simulink model "System_composer__model_pre_alpha_V2"  (R2022b)
settings: Solver=VariableStepAuto  StartTime=0.0  StopTime=10.0  RelTol=1e-3
(part 2 of 3)

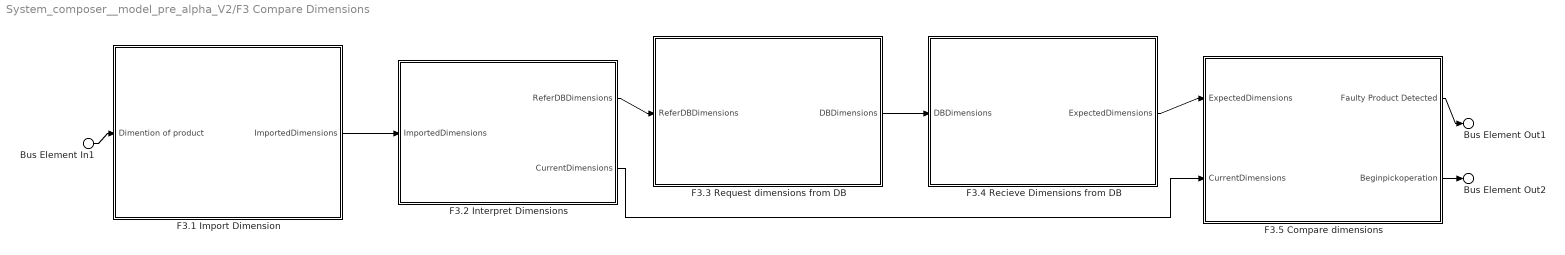
== system System_composer__model_pre_alpha_V2/F3 Compare Dimensions ==
  Bus Element In1 : Inport  PortName=Dimention of product
  F3.1 Import Dimension : Subsystem
      settings: PortSchema="{\"entries\":[{\"content\":{\"headerSize\":26,\"margin\":15,\"minimumSpacing\":25,\"sides\":[{\"content\":{\"connectorIds\":[\"In1\"]},\"type\":\"ConnectorPlacement.EquallySpacedRectSide\",\"uuid\":\"7013333b-bcb0-472a-8b4b-201a684e0f69\"},{\"content\":{\"connectorIds\":[\"Out1\"],\"side\":\"RIGHT\"},\"type\":\"ConnectorPlacement.EquallySpacedRectSide\",\"uuid\":\"4b4cc890-b976-4837-92a8-5b6c4ad3f659\"},{\"content\":{\"connectorIds\":[],\"side\":\"TOP\"},\"type\":\"ConnectorPlacement.EquallySpacedRectSide\",\"uuid\":\"d943cfaa-ae22-4a3b-a19a-c6fb5e90d8f6\"}]},\"type\":\"ConnectorPlacement.EquallySpacedConnector\",\"uuid\":\"02e5c76f-f132-4257-84b4-ea3020272a7a\"}],\"packageUris\":[\"http://schema.mathworks.com/mf0/Connector/R2020b\"],\"version\":\"1.0\"}"
  F3.2 Interpret Dimensions : Subsystem
      settings: PortSchema="{\"entries\":[{\"content\":{\"headerSize\":26,\"margin\":15,\"minimumSpacing\":25,\"sides\":[{\"content\":{\"connectorIds\":[\"In1\"]},\"type\":\"ConnectorPlacement.EquallySpacedRectSide\",\"uuid\":\"7013333b-bcb0-472a-8b4b-201a684e0f69\"},{\"content\":{\"connectorIds\":[\"Out1\",\"Out2\"],\"side\":\"RIGHT\"},\"type\":\"ConnectorPlacement.EquallySpacedRectSide\",\"uuid\":\"4b4cc890-b976-4837-92a8-5b6c4ad3f659\"},{\"content\":{\"connectorIds\":[],\"side\":\"TOP\"},\"type\":\"ConnectorPlacement.EquallySpacedRectSide\",\"uuid\":\"d943cfaa-ae22-4a3b-a19a-c6fb5e90d8f6\"}]},\"type\":\"ConnectorPlacement.EquallySpacedConnector\",\"uuid\":\"02e5c76f-f132-4257-84b4-ea3020272a7a\"}],\"packageUris\":[\"http://schema.mathworks.com/mf0/Connector/R2020b\"],\"version\":\"1.0\"}"
  F3.3 Request dimensions from DB : Subsystem
      settings: PortSchema="{\"entries\":[{\"content\":{\"headerSize\":26,\"margin\":15,\"minimumSpacing\":25,\"sides\":[{\"content\":{\"connectorIds\":[\"In1\"]},\"type\":\"ConnectorPlacement.EquallySpacedRectSide\",\"uuid\":\"7013333b-bcb0-472a-8b4b-201a684e0f69\"},{\"content\":{\"connectorIds\":[\"Out1\"],\"side\":\"RIGHT\"},\"type\":\"ConnectorPlacement.EquallySpacedRectSide\",\"uuid\":\"4b4cc890-b976-4837-92a8-5b6c4ad3f659\"},{\"content\":{\"connectorIds\":[],\"side\":\"TOP\"},\"type\":\"ConnectorPlacement.EquallySpacedRectSide\",\"uuid\":\"d943cfaa-ae22-4a3b-a19a-c6fb5e90d8f6\"}]},\"type\":\"ConnectorPlacement.EquallySpacedConnector\",\"uuid\":\"02e5c76f-f132-4257-84b4-ea3020272a7a\"}],\"packageUris\":[\"http://schema.mathworks.com/mf0/Connector/R2020b\"],\"version\":\"1.0\"}"
  F3.4 Recieve Dimensions from DB : Subsystem
      settings: PortSchema="{\"entries\":[{\"content\":{\"headerSize\":26,\"margin\":15,\"minimumSpacing\":25,\"sides\":[{\"content\":{\"connectorIds\":[\"In1\"]},\"type\":\"ConnectorPlacement.EquallySpacedRectSide\",\"uuid\":\"7013333b-bcb0-472a-8b4b-201a684e0f69\"},{\"content\":{\"connectorIds\":[\"Out1\"],\"side\":\"RIGHT\"},\"type\":\"ConnectorPlacement.EquallySpacedRectSide\",\"uuid\":\"4b4cc890-b976-4837-92a8-5b6c4ad3f659\"},{\"content\":{\"connectorIds\":[],\"side\":\"TOP\"},\"type\":\"ConnectorPlacement.EquallySpacedRectSide\",\"uuid\":\"d943cfaa-ae22-4a3b-a19a-c6fb5e90d8f6\"}]},\"type\":\"ConnectorPlacement.EquallySpacedConnector\",\"uuid\":\"02e5c76f-f132-4257-84b4-ea3020272a7a\"}],\"packageUris\":[\"http://schema.mathworks.com/mf0/Connector/R2020b\"],\"version\":\"1.0\"}"
  F3.5 Compare dimensions : Subsystem
      settings: PortSchema="{\"entries\":[{\"content\":{\"headerSize\":26,\"margin\":15,\"minimumSpacing\":25,\"sides\":[{\"content\":{\"connectorIds\":[\"In1\",\"In2\"]},\"type\":\"ConnectorPlacement.EquallySpacedRectSide\",\"uuid\":\"7013333b-bcb0-472a-8b4b-201a684e0f69\"},{\"content\":{\"connectorIds\":[\"Out1\",\"Out2\"],\"side\":\"RIGHT\"},\"type\":\"ConnectorPlacement.EquallySpacedRectSide\",\"uuid\":\"4b4cc890-b976-4837-92a8-5b6c4ad3f659\"},{\"content\":{\"connectorIds\":[],\"side\":\"TOP\"},\"type\":\"ConnectorPlacement.EquallySpacedRectSide\",\"uuid\":\"d943cfaa-ae22-4a3b-a19a-c6fb5e90d8f6\"}]},\"type\":\"ConnectorPlacement.EquallySpacedConnector\",\"uuid\":\"02e5c76f-f132-4257-84b4-ea3020272a7a\"}],\"packageUris\":[\"http://schema.mathworks.com/mf0/Connector/R2020b\"],\"version\":\"1.0\"}"
  Bus Element Out1 : Outport  PortName=Faulty Product Detected
  Bus Element Out2 : Outport  Port=2  PortName=Beiginpickoperation
  wires:
  F3.5 Compare dimensions/1(Faulty Product Detected) -> Bus Element Out1/1
  F3.3 Request dimensions from DB/1(DBDimensions) -> F3.4 Recieve Dimensions from DB/1(DBDimensions)
  F3.2 Interpret Dimensions/2(CurrentDimensions) -> F3.5 Compare dimensions/2(CurrentDimensions)
  F3.1 Import Dimension/1(ImportedDimensions) -> F3.2 Interpret Dimensions/1(ImportedDimensions)
  Bus Element In1/1 -> F3.1 Import Dimension/1(Dimention of product)
  F3.5 Compare dimensions/2(Beginpickoperation) -> Bus Element Out2/1
  F3.2 Interpret Dimensions/1(ReferDBDimensions) -> F3.3 Request dimensions from DB/1(ReferDBDimensions)
  F3.4 Recieve Dimensions from DB/1(ExpectedDimensions) -> F3.5 Compare dimensions/1(ExpectedDimensions)

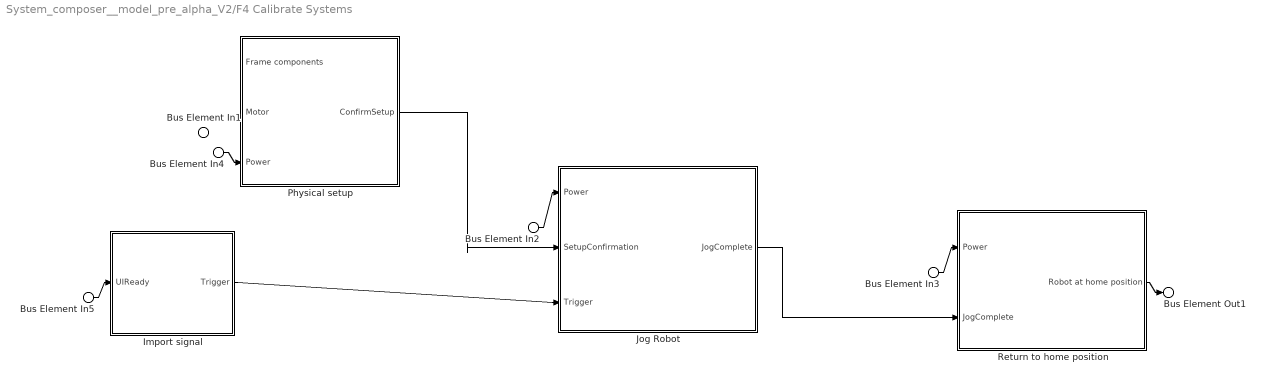
== system System_composer__model_pre_alpha_V2/F4 Calibrate Systems  ==
  Bus Element In1 : Inport  PortName=UIReady
  Bus Element In5 : Inport  PortName=UIReady
  Bus Element In2 : Inport  Port=2  PortName=Power
  Bus Element In3 : Inport  Port=2  PortName=Power
  Bus Element In4 : Inport  Port=2  PortName=Power
  Import signal : Subsystem
      settings: PortSchema="{\"entries\":[{\"content\":{\"headerSize\":26,\"margin\":15,\"minimumSpacing\":25,\"sides\":[{\"content\":{\"connectorIds\":[\"In1\"]},\"type\":\"ConnectorPlacement.EquallySpacedRectSide\",\"uuid\":\"49603a02-1e4e-4380-a56a-8f37f29afafa\"},{\"content\":{\"connectorIds\":[\"Out1\"],\"side\":\"RIGHT\"},\"type\":\"ConnectorPlacement.EquallySpacedRectSide\",\"uuid\":\"ee8e367c-9331-4580-a59d-43baf7bfc40b\"},{\"content\":{\"connectorIds\":[],\"side\":\"TOP\"},\"type\":\"ConnectorPlacement.EquallySpacedRectSide\",\"uuid\":\"fbbd32e3-58f0-4124-8dbd-de003422ef2a\"}]},\"type\":\"ConnectorPlacement.EquallySpacedConnector\",\"uuid\":\"6cb4000c-d9d6-42bd-b109-de2b1ec066aa\"}],\"packageUris\":[\"http://schema.mathworks.com/mf0/Connector/R2020b\"],\"version\":\"1.0\"}"
  Jog Robot : Subsystem
      settings: PortSchema="{\"entries\":[{\"content\":{\"headerSize\":26,\"margin\":15,\"minimumSpacing\":25,\"sides\":[{\"content\":{\"connectorIds\":[\"In1\",\"In2\",\"In3\"]},\"type\":\"ConnectorPlacement.EquallySpacedRectSide\",\"uuid\":\"49603a02-1e4e-4380-a56a-8f37f29afafa\"},{\"content\":{\"connectorIds\":[\"Out1\"],\"side\":\"RIGHT\"},\"type\":\"ConnectorPlacement.EquallySpacedRectSide\",\"uuid\":\"ee8e367c-9331-4580-a59d-43baf7bfc40b\"},{\"content\":{\"connectorIds\":[],\"side\":\"TOP\"},\"type\":\"ConnectorPlacement.EquallySpacedRectSide\",\"uuid\":\"fbbd32e3-58f0-4124-8dbd-de003422ef2a\"}]},\"type\":\"ConnectorPlacement.EquallySpacedConnector\",\"uuid\":\"6cb4000c-d9d6-42bd-b109-de2b1ec066aa\"}],\"packageUris\":[\"http://schema.mathworks.com/mf0/Connector/R2020b\"],\"version\":\"1.0\"}"
  Physical setup : Subsystem
      settings: PortSchema="{\"entries\":[{\"content\":{\"headerSize\":26,\"margin\":15,\"minimumSpacing\":25,\"sides\":[{\"content\":{\"connectorIds\":[\"In1\",\"In2\",\"In3\"]},\"type\":\"ConnectorPlacement.EquallySpacedRectSide\",\"uuid\":\"49603a02-1e4e-4380-a56a-8f37f29afafa\"},{\"content\":{\"connectorIds\":[\"Out1\"],\"side\":\"RIGHT\"},\"type\":\"ConnectorPlacement.EquallySpacedRectSide\",\"uuid\":\"ee8e367c-9331-4580-a59d-43baf7bfc40b\"},{\"content\":{\"connectorIds\":[],\"side\":\"TOP\"},\"type\":\"ConnectorPlacement.EquallySpacedRectSide\",\"uuid\":\"fbbd32e3-58f0-4124-8dbd-de003422ef2a\"}]},\"type\":\"ConnectorPlacement.EquallySpacedConnector\",\"uuid\":\"6cb4000c-d9d6-42bd-b109-de2b1ec066aa\"}],\"packageUris\":[\"http://schema.mathworks.com/mf0/Connector/R2020b\"],\"version\":\"1.0\"}"
  Return to home position : Subsystem
      settings: PortSchema="{\"entries\":[{\"content\":{\"headerSize\":26,\"margin\":15,\"minimumSpacing\":25,\"sides\":[{\"content\":{\"connectorIds\":[\"In1\",\"In2\"]},\"type\":\"ConnectorPlacement.EquallySpacedRectSide\",\"uuid\":\"49603a02-1e4e-4380-a56a-8f37f29afafa\"},{\"content\":{\"connectorIds\":[\"Out1\"],\"side\":\"RIGHT\"},\"type\":\"ConnectorPlacement.EquallySpacedRectSide\",\"uuid\":\"ee8e367c-9331-4580-a59d-43baf7bfc40b\"},{\"content\":{\"connectorIds\":[],\"side\":\"TOP\"},\"type\":\"ConnectorPlacement.EquallySpacedRectSide\",\"uuid\":\"fbbd32e3-58f0-4124-8dbd-de003422ef2a\"}]},\"type\":\"ConnectorPlacement.EquallySpacedConnector\",\"uuid\":\"6cb4000c-d9d6-42bd-b109-de2b1ec066aa\"}],\"packageUris\":[\"http://schema.mathworks.com/mf0/Connector/R2020b\"],\"version\":\"1.0\"}"
  Bus Element Out1 : Outport  PortName=ConfirmCalibration
  wires:
  Bus Element In3/1 -> Return to home position/1(Power)
  Bus Element In4/1 -> Physical setup/3(Power)
  Jog Robot/1(JogComplete) -> Return to home position/2(JogComplete)
  Physical setup/1(ConfirmSetup) -> Jog Robot/2(SetupConfirmation)
  Import signal/1(Trigger) -> Jog Robot/3(Trigger)
  Bus Element In2/1 -> Jog Robot/1(Power)
  Bus Element In5/1 -> Import signal/1(UIReady)
  Return to home position/1(Robot at home position) -> Bus Element Out1/1

== system System_composer__model_pre_alpha_V2/F9 Hold Operations ==
  Bus Element In1 : Inport  PortName=Product Not Detected
  F9.1 Pause Operation : Subsystem
      settings: PortSchema="{\"entries\":[{\"content\":{\"headerSize\":26,\"margin\":15,\"minimumSpacing\":25,\"sides\":[{\"content\":{\"connectorIds\":[\"In1\"]},\"type\":\"ConnectorPlacement.EquallySpacedRectSide\",\"uuid\":\"ee97644e-c9ff-4946-8a58-fee1d557a4ad\"},{\"content\":{\"connectorIds\":[\"Out1\"],\"side\":\"RIGHT\"},\"type\":\"ConnectorPlacement.EquallySpacedRectSide\",\"uuid\":\"e20fd496-d0ba-45f7-949d-94f28912a261\"},{\"content\":{\"connectorIds\":[],\"side\":\"TOP\"},\"type\":\"ConnectorPlacement.EquallySpacedRectSide\",\"uuid\":\"6224eb33-55c0-4770-9979-a18202099dbf\"}]},\"type\":\"ConnectorPlacement.EquallySpacedConnector\",\"uuid\":\"f8ef62f6-ad53-4f25-bdc3-ef7ca131dedb\"}],\"packageUris\":[\"http://schema.mathworks.com/mf0/Connector/R2020b\"],\"version\":\"1.0\"}"
  Conn1 : PMIOPort  Side=Left
  Bus Element Out1 : Outport  PortName=Return To Detection
  wires:
  Bus Element In1/1 -> F9.1 Pause Operation/1(Product Not Detected)
  F9.1 Pause Operation/1(Return To Detection) -> Bus Element Out1/1

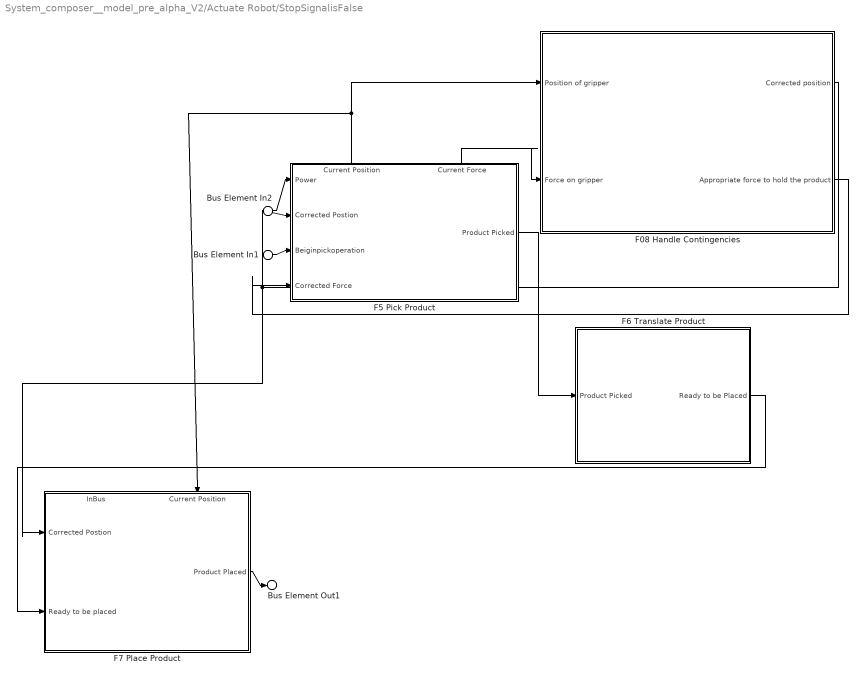
== system System_composer__model_pre_alpha_V2/Actuate Robot/StopSignalisFalse ==
  Bus Element In2 : Inport  PortName=Power
  Bus Element In1 : Inport  Port=2  PortName=Beiginpickoperation
  F08 Handle Contingencies : Subsystem
      settings: PortSchema="{\"entries\":[{\"content\":{\"headerSize\":26,\"margin\":15,\"minimumSpacing\":25,\"sides\":[{\"content\":{\"connectorIds\":[\"In1\",\"In2\"]},\"type\":\"ConnectorPlacement.EquallySpacedRectSide\",\"uuid\":\"1c117138-a6d4-4ec0-b7b8-6d1428745998\"},{\"content\":{\"connectorIds\":[\"Out1\",\"Out2\"],\"side\":\"RIGHT\"},\"type\":\"ConnectorPlacement.EquallySpacedRectSide\",\"uuid\":\"426d6ceb-18a6-42d8-9bd7-8fe69cb751f0\"},{\"content\":{\"connectorIds\":[],\"side\":\"TOP\"},\"type\":\"ConnectorPlacement.EquallySpacedRectSide\",\"uuid\":\"23012487-78cd-45b9-9306-44393710ac2e\"}]},\"type\":\"ConnectorPlacement.EquallySpacedConnector\",\"uuid\":\"f4468a7a-13e2-43af-b621-864ee5d109de\"}],\"packageUris\":[\"http://schema.mathworks.com/mf0/Connector/R2020b\"],\"version\":\"1.0\"}"
  F5 Pick Product : Subsystem
      settings: PortSchema="{\"entries\":[{\"content\":{\"headerSize\":26,\"margin\":15,\"minimumSpacing\":25,\"sides\":[{\"content\":{\"connectorIds\":[\"In1\",\"In2\",\"In3\",\"In4\"]},\"type\":\"ConnectorPlacement.EquallySpacedRectSide\",\"uuid\":\"ce520cb7-ac6b-49f5-959a-43d0066e6af8\"},{\"content\":{\"connectorIds\":[\"Out3\"],\"side\":\"RIGHT\"},\"type\":\"ConnectorPlacement.EquallySpacedRectSide\",\"uuid\":\"785c5fb5-eec3-4a9f-be3c-47cdb1865e9b\"},{\"content\":{\"connectorIds\":[\"Out1\",\"Out2\"],\"side\":\"TOP\"},\"type\":\"ConnectorPlacement.EquallySpacedRectSide\",\"uuid\":\"de1fb606-e36e-4d03-b808-745512e6c407\"}]},\"type\":\"ConnectorPlacement.EquallySpacedConnector\",\"uuid\":\"f62687dc-336d-43b3-90e2-c71aecc80de5\"}],\"packageUris\":[\"http://schema.mathworks.com/mf0/Connector/R2020b\"],\"version\":\"1.0\"}"
  F6 Translate Product : Subsystem
      settings: PortSchema="{\"entries\":[{\"content\":{\"headerSize\":26,\"margin\":15,\"minimumSpacing\":25,\"sides\":[{\"content\":{\"connectorIds\":[\"In1\"]},\"type\":\"ConnectorPlacement.EquallySpacedRectSide\",\"uuid\":\"ce520cb7-ac6b-49f5-959a-43d0066e6af8\"},{\"content\":{\"connectorIds\":[\"Out1\"],\"side\":\"RIGHT\"},\"type\":\"ConnectorPlacement.EquallySpacedRectSide\",\"uuid\":\"785c5fb5-eec3-4a9f-be3c-47cdb1865e9b\"},{\"content\":{\"connectorIds\":[],\"side\":\"TOP\"},\"type\":\"ConnectorPlacement.EquallySpacedRectSide\",\"uuid\":\"de1fb606-e36e-4d03-b808-745512e6c407\"}]},\"type\":\"ConnectorPlacement.EquallySpacedConnector\",\"uuid\":\"f62687dc-336d-43b3-90e2-c71aecc80de5\"}],\"packageUris\":[\"http://schema.mathworks.com/mf0/Connector/R2020b\"],\"version\":\"1.0\"}"
  F7 Place Product : Subsystem
      settings: PortSchema="{\"entries\":[{\"content\":{\"headerSize\":26,\"margin\":15,\"minimumSpacing\":25,\"sides\":[{\"content\":{\"connectorIds\":[\"In4\",\"In3\"]},\"type\":\"ConnectorPlacement.EquallySpacedRectSide\",\"uuid\":\"ce520cb7-ac6b-49f5-959a-43d0066e6af8\"},{\"content\":{\"connectorIds\":[\"Out1\"],\"side\":\"RIGHT\"},\"type\":\"ConnectorPlacement.EquallySpacedRectSide\",\"uuid\":\"785c5fb5-eec3-4a9f-be3c-47cdb1865e9b\"},{\"content\":{\"connectorIds\":[\"In1\",\"In2\"],\"side\":\"TOP\"},\"type\":\"ConnectorPlacement.EquallySpacedRectSide\",\"uuid\":\"de1fb606-e36e-4d03-b808-745512e6c407\"}]},\"type\":\"ConnectorPlacement.EquallySpacedConnector\",\"uuid\":\"f62687dc-336d-43b3-90e2-c71aecc80de5\"}],\"packageUris\":[\"http://schema.mathworks.com/mf0/Connector/R2020b\"],\"version\":\"1.0\"}"
  Bus Element Out1 : Outport  PortName=Product Placed
  wires:
  F6 Translate Product/1(Ready to be Placed) -> F7 Place Product/3(Ready to be placed)
  F5 Pick Product/3(Product Picked) -> F6 Translate Product/1(Product Picked)
  F5 Pick Product/1(Current Position) -> F7 Place Product/2(Current Position), F08 Handle Contingencies/1(Position of gripper)
  F08 Handle Contingencies/1(Corrected position) -> F7 Place Product/4(Corrected Postion), F5 Pick Product/2(Corrected Postion)
  F5 Pick Product/2(Current Force) -> F08 Handle Contingencies/2(Force on gripper)
  F08 Handle Contingencies/2(Appropriate force to hold the product) -> F5 Pick Product/4(Corrected Force)
  Bus Element In1/1 -> F5 Pick Product/3(Beiginpickoperation)
  Bus Element In2/1 -> F5 Pick Product/1(Power)
  F7 Place Product/1(Product Placed) -> Bus Element Out1/1

== system System_composer__model_pre_alpha_V2/Actuate Robot/StopSignalisTrue ==
  Bus Element In1 : Inport  PortName=Stop Signal
  Bus Element Out1 : Outport  PortName=NotifySTOPStatus

== system System_composer__model_pre_alpha_V2/F1 Detect Product/F1.1 Confirm System Calibration ==
  Bus Element In2 : Inport  PortName=ConfirmCalibration
  Bus Element Out1 : Outport  PortName=SystemCallibrated

== system System_composer__model_pre_alpha_V2/F1 Detect Product/F1.2 import signal ==
  Bus Element In5 : Inport  PortName=SystemCallibrated
  Bus Element In4 : Inport  Port=2  PortName=Lookforproduct
  Bus Element In3 : Inport  Port=3  PortName=Reset signal
  Bus Element Out1 : Outport  PortName=InterpretSignal

== system System_composer__model_pre_alpha_V2/F1 Detect Product/F1.3 Sense Product ==
  Bus Element In2 : Inport  PortName=Product
  Bus Element In1 : Inport  Port=2  PortName=InterpretSignal
  Bus Element Out2 : Outport  PortName=Product Detected
  Bus Element Out1 : Outport  Port=2  PortName=Count
  Bus Element Out3 : Outport  Port=3  PortName=ProductNOTdetected

== system System_composer__model_pre_alpha_V2/F10 Halt Operations/F10.1 Recieve Button Input ==
  Bus Element In1 : Inport  PortName=EmergencyStopSignal
  Bus Element Out1 : Outport  PortName=RecievedInput

== system System_composer__model_pre_alpha_V2/F10 Halt Operations/F10.2 Interpret Input ==
  Bus Element In1 : Inport  PortName=RecievedInput
  Bus Element Out1 : Outport  PortName=StopOperation

== system System_composer__model_pre_alpha_V2/F10 Halt Operations/F10.3 Stop Actuators ==
  Bus Element In1 : Inport  PortName=StopOperation
  Bus Element Out2 : Outport  PortName=NotifyOperator
  Bus Element Out1 : Outport  Port=2  PortName=Stop Signal

== system System_composer__model_pre_alpha_V2/F10 Halt Operations/F10.4 Export Signal ==
  Bus Element In1 : Inport  PortName=NotifyOperator
  Bus Element Out1 : Outport  PortName=NotifySTOP

== system System_composer__model_pre_alpha_V2/F11 Handle User Interface/F 11.1Notify user (Logout Successful) ==
  Bus Element In1 : Inport  PortName=ResetConfirm
  Bus Element Out1 : Outport  PortName=Logout Successful

== system System_composer__model_pre_alpha_V2/F11 Handle User Interface/F11.10 Monitor System Parameters ==
  Bus Element In2 : Inport  PortName=Stop Button
  Bus Element In1 : Inport  Port=2  PortName=DashboardLoaded
  Bus Element In3 : Inport  Port=3  PortName=Faulty Product Detected
  Bus Element In5 : Inport  Port=4  PortName=observeparameters
  Bus Element In4 : Inport  Port=5  PortName=Count
  Bus Element Out2 : Outport  PortName=NotifyEmergency
  Bus Element Out1 : Outport  Port=2  PortName=ShowParameters

== system System_composer__model_pre_alpha_V2/F11 Handle User Interface/F11.11 Notify User ==
  Bus Element In1 : Inport  PortName=NotifyEmergency

== system System_composer__model_pre_alpha_V2/F11 Handle User Interface/F11.12Confirm System STOP ==
  Bus Element In1 : Inport  PortName=LOGOUTConfirm
  Bus Element In2 : Inport  Port=2  PortName=STOPConfirm
  Bus Element Out1 : Outport  PortName=Resetsystem

== system System_composer__model_pre_alpha_V2/F11 Handle User Interface/F11.13 Generate STOP Signal ==
  Bus Element In1 : Inport  PortName=DBUpdated
  Bus Element Out1 : Outport  PortName=STOPoperation

== system System_composer__model_pre_alpha_V2/F11 Handle User Interface/F11.14 Update Activity Log ==
  Bus Element In1 : Inport  PortName=LogoutPrompt
  Bus Element Out1 : Outport  PortName=LOGOUTConfirm
  Bus Element Out2 : Outport  Port=2  PortName=DBUpdated

== system System_composer__model_pre_alpha_V2/F11 Handle User Interface/F11.15 Display System Parameters ==
  Bus Element In1 : Inport  PortName=ShowParameters
  Bus Element Out4 : Outport  PortName=SystemState
  Bus Element Out3 : Outport  Port=2  PortName=LogoutPrompt
  Bus Element Out2 : Outport  Port=3  PortName=observeparameters

== system System_composer__model_pre_alpha_V2/F11 Handle User Interface/F11.2 Turn ON System ==
  Bus Element In1 : Inport  PortName=Power Supply
  Bus Element Out1 : Outport  PortName=WaitforInput

== system System_composer__model_pre_alpha_V2/F11 Handle User Interface/F11.3 Recieve User Input ==
  Bus Element In1 : Inport  PortName=WaitforInput
  Bus Element In2 : Inport  Port=2  PortName=User Input
  Bus Element Out1 : Outport  PortName=ReadytoInteract

== system System_composer__model_pre_alpha_V2/F11 Handle User Interface/F11.4 Provide User Interface ==
  Bus Element In1 : Inport  PortName=ReadytoInteract
  Bus Element Out1 : Outport  PortName=VisualsReady

== system System_composer__model_pre_alpha_V2/F11 Handle User Interface/F11.5 Recieve Credentials ==
  Bus Element In1 : Inport  PortName=VisualsReady
  Bus Element In2 : Inport  Port=2  PortName=User Credentials
  Bus Element Out1 : Outport  PortName=RecievedCredentials

== system System_composer__model_pre_alpha_V2/F11 Handle User Interface/F11.6 Verify Credentials ==
  Bus Element In1 : Inport  PortName=RecievedCredentials
  Bus Element Out1 : Outport  PortName=Confirmation

== system System_composer__model_pre_alpha_V2/F11 Handle User Interface/F11.7 Confirm Login ==
  Bus Element In1 : Inport  PortName=Confirmation
  Bus Element Out2 : Outport  PortName=LOGINConfirm
  Bus Element Out1 : Outport  Port=2  PortName=OpenDashboard

== system System_composer__model_pre_alpha_V2/F11 Handle User Interface/F11.8 Provide System Dashboard ==
  Bus Element In1 : Inport  PortName=OpenDashboard
  Bus Element Out1 : Outport  PortName=DashboardLoaded

== system System_composer__model_pre_alpha_V2/F12 Reset Position/F12.1 Obtain the coordinates of home position ==
  Bus Element In1 : Inport  PortName=Product placed
  Bus Element In2 : Inport  Port=2  PortName=Log-out
  Bus Element Out1 : Outport  PortName=home position

== system System_composer__model_pre_alpha_V2/F12 Reset Position/F12.2 Go to home ==
  Bus Element In1 : Inport  PortName=home position
  Bus Element Out2 : Outport  PortName=Coordinates
  Bus Element Out1 : Outport  Port=2  PortName=power off signal

== system System_composer__model_pre_alpha_V2/F12 Reset Position/F12.3 Freeze the actuators ==
  Bus Element In1 : Inport  PortName=power off signal
  Bus Element Out1 : Outport  PortName=System ready

== system System_composer__model_pre_alpha_V2/F12 Reset Position/F12.4Hold the end effector at home position ==
  Bus Element In1 : Inport  PortName=Coordinates

== system System_composer__model_pre_alpha_V2/F2 Inspect Product/Capture image of product ==
  Bus Element In2 : Inport  PortName=Product
  Bus Element In1 : Inport  Port=2  PortName=Power
  Bus Element In3 : Inport  Port=3  PortName=Trigger
  Bus Element Out3 : Outport  PortName=ProductImage
  Bus Element Out1 : Outport  Port=2  PortName=OutBus1
  Bus Element Out2 : Outport  Port=3  PortName=OutBus

== system System_composer__model_pre_alpha_V2/F2 Inspect Product/Compute dimentions of product ==
  Bus Element In1 : Inport  PortName=Product image
  Compute dimention : Subsystem
      settings: PortSchema="{\"entries\":[{\"content\":{\"headerSize\":26,\"margin\":15,\"minimumSpacing\":25,\"sides\":[{\"content\":{\"connectorIds\":[\"In1\"]},\"type\":\"ConnectorPlacement.EquallySpacedRectSide\",\"uuid\":\"320e88d4-3d78-4d2f-ad02-b343723442c4\"},{\"content\":{\"connectorIds\":[\"Out1\"],\"side\":\"RIGHT\"},\"type\":\"ConnectorPlacement.EquallySpacedRectSide\",\"uuid\":\"09c33032-32ab-4ada-8ed8-0201f1b57dc0\"},{\"content\":{\"connectorIds\":[],\"side\":\"TOP\"},\"type\":\"ConnectorPlacement.EquallySpacedRectSide\",\"uuid\":\"2b028b26-f15f-43e2-ad75-04cde6dc5293\"}]},\"type\":\"ConnectorPlacement.EquallySpacedConnector\",\"uuid\":\"3dd2f29f-a920-492f-a094-d6d7756d0428\"}],\"packageUris\":[\"http://schema.mathworks.com/mf0/Connector/R2020b\"],\"version\":\"1.0\"}"
  get coordinates : Subsystem
      settings: PortSchema="{\"entries\":[{\"content\":{\"headerSize\":26,\"margin\":15,\"minimumSpacing\":25,\"sides\":[{\"content\":{\"connectorIds\":[\"In1\"]},\"type\":\"ConnectorPlacement.EquallySpacedRectSide\",\"uuid\":\"320e88d4-3d78-4d2f-ad02-b343723442c4\"},{\"content\":{\"connectorIds\":[\"Out1\"],\"side\":\"RIGHT\"},\"type\":\"ConnectorPlacement.EquallySpacedRectSide\",\"uuid\":\"09c33032-32ab-4ada-8ed8-0201f1b57dc0\"},{\"content\":{\"connectorIds\":[],\"side\":\"TOP\"},\"type\":\"ConnectorPlacement.EquallySpacedRectSide\",\"uuid\":\"2b028b26-f15f-43e2-ad75-04cde6dc5293\"}]},\"type\":\"ConnectorPlacement.EquallySpacedConnector\",\"uuid\":\"3dd2f29f-a920-492f-a094-d6d7756d0428\"}],\"packageUris\":[\"http://schema.mathworks.com/mf0/Connector/R2020b\"],\"version\":\"1.0\"}"
  Bus Element Out1 : Outport  PortName=Dimention of product
  wires:
  Bus Element In1/1 -> get coordinates/1(Product image)
  get coordinates/1(Coordinates) -> Compute dimention/1(Coordinates)
  Compute dimention/1(Dimention of product) -> Bus Element Out1/1

== system System_composer__model_pre_alpha_V2/F2 Inspect Product/Detect QR Code ==
  Bus Element In1 : Inport  PortName=ProductImage
  Bus Element Out1 : Outport  PortName=ExtractedQRCode

== system System_composer__model_pre_alpha_V2/F2 Inspect Product/Export Orientation ==
  Bus Element In1 : Inport  PortName=Product image
  Bus Element Out1 : Outport  PortName=ProductOrientation

== system System_composer__model_pre_alpha_V2/F2 Inspect Product/Import QR Code ==
  Bus Element In1 : Inport  PortName=ExtractedQRCOde
  Bus Element Out1 : Outport  PortName=ExportQR

== system System_composer__model_pre_alpha_V2/F2 Inspect Product/Import product ==
  Bus Element In1 : Inport  PortName=Product
  Bus Element Out1 : Outport  PortName=OutBus

== system System_composer__model_pre_alpha_V2/F2 Inspect Product/Import signal ==
  Bus Element In1 : Inport  PortName=Detection signal
  Bus Element Out1 : Outport  PortName=Trigger

== system System_composer__model_pre_alpha_V2/F2 Inspect Product/Record position of Product ==
  Bus Element In1 : Inport  PortName=Product image
  Bus Element Out1 : Outport  PortName=ProductPosition

== system System_composer__model_pre_alpha_V2/F3 Compare Dimensions/F3.1 Import Dimension ==
  Bus Element In1 : Inport  PortName=Dimention of product
  Bus Element Out1 : Outport  PortName=ImportedDimensions

== system System_composer__model_pre_alpha_V2/F3 Compare Dimensions/F3.2 Interpret Dimensions ==
  Bus Element In1 : Inport  PortName=ImportedDimensions
  Bus Element Out1 : Outport  PortName=ReferDBDimensions
  Bus Element Out2 : Outport  Port=2  PortName=CurrentDimensions

== system System_composer__model_pre_alpha_V2/F3 Compare Dimensions/F3.3 Request dimensions from DB ==
  Bus Element In1 : Inport  PortName=ReferDBDimensions
  Bus Element Out1 : Outport  PortName=DBDimensions

== system System_composer__model_pre_alpha_V2/F3 Compare Dimensions/F3.4 Recieve Dimensions from DB ==
  Bus Element In1 : Inport  PortName=DBDimensions
  Bus Element Out1 : Outport  PortName=ExpectedDimensions

== system System_composer__model_pre_alpha_V2/F3 Compare Dimensions/F3.5 Compare dimensions ==
  Bus Element In2 : Inport  PortName=ExpectedDimensions
  Bus Element In1 : Inport  Port=2  PortName=CurrentDimensions
  Bus Element Out1 : Outport  PortName=Faulty Product Detected
  Bus Element Out2 : Outport  Port=2  PortName=Beginpickoperation

== system System_composer__model_pre_alpha_V2/F4 Calibrate Systems /Import signal ==
  Bus Element In1 : Inport  PortName=UIReady
  Bus Element Out1 : Outport  PortName=Trigger

== system System_composer__model_pre_alpha_V2/F4 Calibrate Systems /Jog Robot ==
  Bus Element In1 : Inport  PortName=Power
  Bus Element In2 : Inport  Port=2  PortName=SetupConfirmation
  Bus Element In3 : Inport  Port=3  PortName=Trigger
  Bus Element Out1 : Outport  PortName=JogComplete

== system System_composer__model_pre_alpha_V2/F4 Calibrate Systems /Physical setup ==
  Bus Element In1 : Inport  PortName=Frame components
  Bus Element In2 : Inport  Port=2  PortName=Motor
  Bus Element In3 : Inport  Port=3  PortName=Power
  Frame setup : Subsystem
      settings: PortSchema="{\"entries\":[{\"content\":{\"headerSize\":26,\"margin\":15,\"minimumSpacing\":25,\"sides\":[{\"content\":{\"connectorIds\":[\"In1\"]},\"type\":\"ConnectorPlacement.EquallySpacedRectSide\",\"uuid\":\"49603a02-1e4e-4380-a56a-8f37f29afafa\"},{\"content\":{\"connectorIds\":[\"Out1\"],\"side\":\"RIGHT\"},\"type\":\"ConnectorPlacement.EquallySpacedRectSide\",\"uuid\":\"ee8e367c-9331-4580-a59d-43baf7bfc40b\"},{\"content\":{\"connectorIds\":[],\"side\":\"TOP\"},\"type\":\"ConnectorPlacement.EquallySpacedRectSide\",\"uuid\":\"fbbd32e3-58f0-4124-8dbd-de003422ef2a\"}]},\"type\":\"ConnectorPlacement.EquallySpacedConnector\",\"uuid\":\"6cb4000c-d9d6-42bd-b109-de2b1ec066aa\"}],\"packageUris\":[\"http://schema.mathworks.com/mf0/Connector/R2020b\"],\"version\":\"1.0\"}"
  Motor setup : Subsystem
      settings: PortSchema="{\"entries\":[{\"content\":{\"headerSize\":26,\"margin\":15,\"minimumSpacing\":25,\"sides\":[{\"content\":{\"connectorIds\":[\"In1\",\"In2\"]},\"type\":\"ConnectorPlacement.EquallySpacedRectSide\",\"uuid\":\"49603a02-1e4e-4380-a56a-8f37f29afafa\"},{\"content\":{\"connectorIds\":[\"Out1\"],\"side\":\"RIGHT\"},\"type\":\"ConnectorPlacement.EquallySpacedRectSide\",\"uuid\":\"ee8e367c-9331-4580-a59d-43baf7bfc40b\"},{\"content\":{\"connectorIds\":[],\"side\":\"TOP\"},\"type\":\"ConnectorPlacement.EquallySpacedRectSide\",\"uuid\":\"fbbd32e3-58f0-4124-8dbd-de003422ef2a\"}]},\"type\":\"ConnectorPlacement.EquallySpacedConnector\",\"uuid\":\"6cb4000c-d9d6-42bd-b109-de2b1ec066aa\"}],\"packageUris\":[\"http://schema.mathworks.com/mf0/Connector/R2020b\"],\"version\":\"1.0\"}"
  Power upset : Subsystem
      settings: PortSchema="{\"entries\":[{\"content\":{\"headerSize\":26,\"margin\":15,\"minimumSpacing\":25,\"sides\":[{\"content\":{\"connectorIds\":[\"In1\",\"In2\"]},\"type\":\"ConnectorPlacement.EquallySpacedRectSide\",\"uuid\":\"49603a02-1e4e-4380-a56a-8f37f29afafa\"},{\"content\":{\"connectorIds\":[\"Out1\"],\"side\":\"RIGHT\"},\"type\":\"ConnectorPlacement.EquallySpacedRectSide\",\"uuid\":\"ee8e367c-9331-4580-a59d-43baf7bfc40b\"},{\"content\":{\"connectorIds\":[],\"side\":\"TOP\"},\"type\":\"ConnectorPlacement.EquallySpacedRectSide\",\"uuid\":\"fbbd32e3-58f0-4124-8dbd-de003422ef2a\"}]},\"type\":\"ConnectorPlacement.EquallySpacedConnector\",\"uuid\":\"6cb4000c-d9d6-42bd-b109-de2b1ec066aa\"}],\"packageUris\":[\"http://schema.mathworks.com/mf0/Connector/R2020b\"],\"version\":\"1.0\"}"
  Bus Element Out1 : Outport  PortName=ConfirmSetup
  wires:
  Bus Element In1/1 -> Frame setup/1(Frame components)
  Frame setup/1(Frame) -> Motor setup/1(Frame)
  Motor setup/1(Frame and motor setup) -> Power upset/2(Frame and motor setup)
  Bus Element In2/1 -> Motor setup/2(Motor)
  Bus Element In3/1 -> Power upset/1(Power)
  Power upset/1(Physical setup) -> Bus Element Out1/1

== system System_composer__model_pre_alpha_V2/F4 Calibrate Systems /Return to home position ==
  Bus Element In2 : Inport  PortName=Power
  Bus Element In1 : Inport  Port=2  PortName=JogComplete
  Bus Element Out1 : Outport  PortName=Robot at home position

== system System_composer__model_pre_alpha_V2/F9 Hold Operations/F9.1 Pause Operation ==
  Bus Element In1 : Inport  PortName=Product Not Detected
  Bus Element Out1 : Outport  PortName=Return To Detection

== system System_composer__model_pre_alpha_V2/Actuate Robot/StopSignalisFalse/F08 Handle Contingencies ==
  In Bus Element : Inport  PortName=Position of gripper
  In Bus Element1 : Inport  Port=2  PortName=Force on gripper
  Check Pick Position : Subsystem  Variant=on  VariantControlMode=label  LabelModeActiveChoice=true
      settings: PortSchema="{\"entries\":[{\"content\":{\"headerSize\":38,\"margin\":15,\"minimumSpacing\":25,\"sides\":[{\"content\":{\"connectorIds\":[\"In1\"]},\"type\":\"ConnectorPlacement.EquallySpacedRectSide\",\"uuid\":\"82248304-a162-48ca-a47b-1ca98baf0c4b\"},{\"content\":{\"connectorIds\":[\"Out1\"],\"side\":\"RIGHT\"},\"type\":\"ConnectorPlacement.EquallySpacedRectSide\",\"uuid\":\"4a71fcf9-75ca-4fc2-a495-265b9c18be6e\"},{\"content\":{\"connectorIds\":[],\"side\":\"TOP\"},\"type\":\"ConnectorPlacement.EquallySpacedRectSide\",\"uuid\":\"a8916134-5d81-43cb-b01e-b135fd95b202\"}]},\"type\":\"ConnectorPlacement.EquallySpacedConnector\",\"uuid\":\"0453f589-d612-429d-a4fd-aaf4ba456e8c\"}],\"packageUris\":[\"http://schema.mathworks.com/mf0/Connector/R2020b\"],\"version\":\"1.0\"}"
  F8.1Weak force on the product : Subsystem
      settings: PortSchema="{\"entries\":[{\"content\":{\"headerSize\":26,\"margin\":15,\"minimumSpacing\":25,\"sides\":[{\"content\":{\"connectorIds\":[\"In1\"]},\"type\":\"ConnectorPlacement.EquallySpacedRectSide\",\"uuid\":\"cfa9a458-ccb1-4b4b-9223-cdb6aaef5fc4\"},{\"content\":{\"connectorIds\":[\"Out1\"],\"side\":\"RIGHT\"},\"type\":\"ConnectorPlacement.EquallySpacedRectSide\",\"uuid\":\"f9e6f688-270f-46a5-8c07-32c6831cf3d3\"},{\"content\":{\"connectorIds\":[],\"side\":\"TOP\"},\"type\":\"ConnectorPlacement.EquallySpacedRectSide\",\"uuid\":\"2fcd258a-a10a-44a0-bcb2-682252ae81b0\"}]},\"type\":\"ConnectorPlacement.EquallySpacedConnector\",\"uuid\":\"80e45476-3fa2-42b9-aef1-d9f502108577\"}],\"packageUris\":[\"http://schema.mathworks.com/mf0/Connector/R2020b\"],\"version\":\"1.0\"}"
  Out Bus Element1 : Outport  PortName=Corrected position
  Out Bus Element : Outport  Port=2  PortName=Appropriate force to hold the product
  wires:
  In Bus Element1/1 -> F8.1Weak force on the product/1(Force on gripper)
  In Bus Element/1 -> Check Pick Position/1(Position of gripper)
  Check Pick Position/1(Corrected position) -> Out Bus Element1/1
  F8.1Weak force on the product/1(Appropriate force) -> Out Bus Element/1

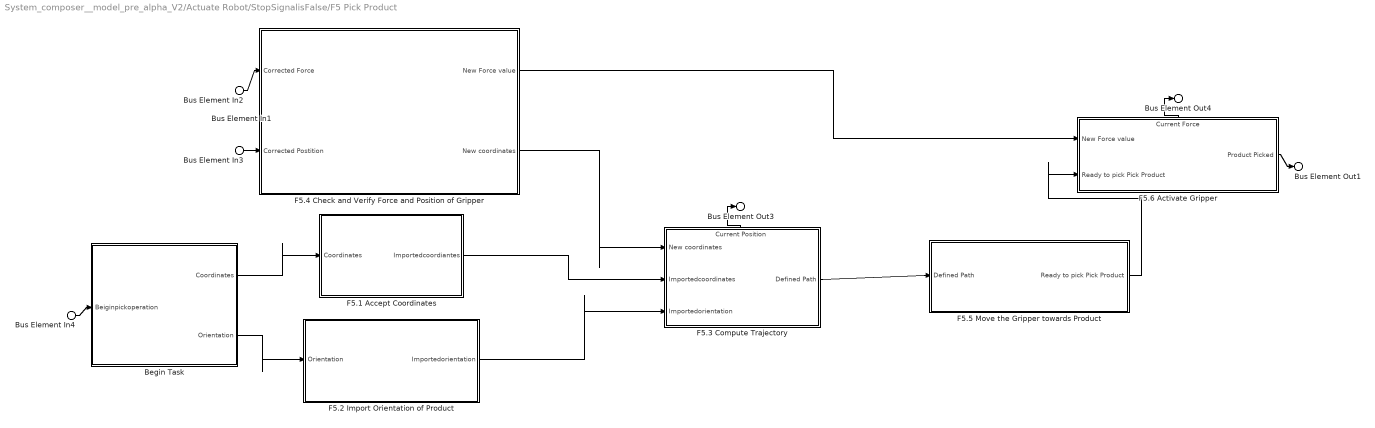
== system System_composer__model_pre_alpha_V2/Actuate Robot/StopSignalisFalse/F5 Pick Product ==
  Bus Element In1 : Inport  PortName=Power
  Bus Element In2 : Inport  Port=2  PortName=Corrected Postion
  Bus Element In4 : Inport  Port=3  PortName=Beiginpickoperation
  Bus Element In3 : Inport  Port=4  PortName=Corrected Force
  Begin Task : Subsystem
      settings: PortSchema="{\"entries\":[{\"content\":{\"headerSize\":26,\"margin\":15,\"minimumSpacing\":25,\"sides\":[{\"content\":{\"connectorIds\":[\"In1\"]},\"type\":\"ConnectorPlacement.EquallySpacedRectSide\",\"uuid\":\"ae240f5f-39ed-41a3-b9a8-bf2f33b986be\"},{\"content\":{\"connectorIds\":[\"Out1\",\"Out2\"],\"side\":\"RIGHT\"},\"type\":\"ConnectorPlacement.EquallySpacedRectSide\",\"uuid\":\"44ba199a-fd12-4621-8565-f3f1adedec4a\"},{\"content\":{\"connectorIds\":[],\"side\":\"TOP\"},\"type\":\"ConnectorPlacement.EquallySpacedRectSide\",\"uuid\":\"41d301d8-0f91-4ed1-b07b-750dd04e1ae2\"}]},\"type\":\"ConnectorPlacement.EquallySpacedConnector\",\"uuid\":\"8d081691-644b-416f-87ea-d7e0a52b2ce6\"}],\"packageUris\":[\"http://schema.mathworks.com/mf0/Connector/R2020b\"],\"version\":\"1.0\"}"
  F5.1 Accept Coordinates : Subsystem
      settings: PortSchema="{\"entries\":[{\"content\":{\"headerSize\":26,\"margin\":15,\"minimumSpacing\":25,\"sides\":[{\"content\":{\"connectorIds\":[\"In1\"]},\"type\":\"ConnectorPlacement.EquallySpacedRectSide\",\"uuid\":\"ce520cb7-ac6b-49f5-959a-43d0066e6af8\"},{\"content\":{\"connectorIds\":[\"Out1\"],\"side\":\"RIGHT\"},\"type\":\"ConnectorPlacement.EquallySpacedRectSide\",\"uuid\":\"785c5fb5-eec3-4a9f-be3c-47cdb1865e9b\"},{\"content\":{\"connectorIds\":[],\"side\":\"TOP\"},\"type\":\"ConnectorPlacement.EquallySpacedRectSide\",\"uuid\":\"de1fb606-e36e-4d03-b808-745512e6c407\"}]},\"type\":\"ConnectorPlacement.EquallySpacedConnector\",\"uuid\":\"f62687dc-336d-43b3-90e2-c71aecc80de5\"}],\"packageUris\":[\"http://schema.mathworks.com/mf0/Connector/R2020b\"],\"version\":\"1.0\"}"
  F5.2 Import Orientation of Product : Subsystem
      settings: PortSchema="{\"entries\":[{\"content\":{\"headerSize\":26,\"margin\":15,\"minimumSpacing\":25,\"sides\":[{\"content\":{\"connectorIds\":[\"In1\"]},\"type\":\"ConnectorPlacement.EquallySpacedRectSide\",\"uuid\":\"ce520cb7-ac6b-49f5-959a-43d0066e6af8\"},{\"content\":{\"connectorIds\":[\"Out1\"],\"side\":\"RIGHT\"},\"type\":\"ConnectorPlacement.EquallySpacedRectSide\",\"uuid\":\"785c5fb5-eec3-4a9f-be3c-47cdb1865e9b\"},{\"content\":{\"connectorIds\":[],\"side\":\"TOP\"},\"type\":\"ConnectorPlacement.EquallySpacedRectSide\",\"uuid\":\"de1fb606-e36e-4d03-b808-745512e6c407\"}]},\"type\":\"ConnectorPlacement.EquallySpacedConnector\",\"uuid\":\"f62687dc-336d-43b3-90e2-c71aecc80de5\"}],\"packageUris\":[\"http://schema.mathworks.com/mf0/Connector/R2020b\"],\"version\":\"1.0\"}"
  F5.3 Compute Trajectory : Subsystem
      settings: PortSchema="{\"entries\":[{\"content\":{\"headerSize\":26,\"margin\":15,\"minimumSpacing\":25,\"sides\":[{\"content\":{\"connectorIds\":[\"In1\",\"In2\",\"In3\"]},\"type\":\"ConnectorPlacement.EquallySpacedRectSide\",\"uuid\":\"ce520cb7-ac6b-49f5-959a-43d0066e6af8\"},{\"content\":{\"connectorIds\":[\"Out2\"],\"side\":\"RIGHT\"},\"type\":\"ConnectorPlacement.EquallySpacedRectSide\",\"uuid\":\"785c5fb5-eec3-4a9f-be3c-47cdb1865e9b\"},{\"content\":{\"connectorIds\":[\"Out1\"],\"side\":\"TOP\"},\"type\":\"ConnectorPlacement.EquallySpacedRectSide\",\"uuid\":\"de1fb606-e36e-4d03-b808-745512e6c407\"}]},\"type\":\"ConnectorPlacement.EquallySpacedConnector\",\"uuid\":\"f62687dc-336d-43b3-90e2-c71aecc80de5\"}],\"packageUris\":[\"http://schema.mathworks.com/mf0/Connector/R2020b\"],\"version\":\"1.0\"}"
  F5.4 Check and Verify Force and Position of Gripper : Subsystem
      settings: PortSchema="{\"entries\":[{\"content\":{\"headerSize\":26,\"margin\":15,\"minimumSpacing\":25,\"sides\":[{\"content\":{\"connectorIds\":[\"In1\",\"In2\"]},\"type\":\"ConnectorPlacement.EquallySpacedRectSide\",\"uuid\":\"ce520cb7-ac6b-49f5-959a-43d0066e6af8\"},{\"content\":{\"connectorIds\":[\"Out1\",\"Out2\"],\"side\":\"RIGHT\"},\"type\":\"ConnectorPlacement.EquallySpacedRectSide\",\"uuid\":\"785c5fb5-eec3-4a9f-be3c-47cdb1865e9b\"},{\"content\":{\"connectorIds\":[],\"side\":\"TOP\"},\"type\":\"ConnectorPlacement.EquallySpacedRectSide\",\"uuid\":\"de1fb606-e36e-4d03-b808-745512e6c407\"},{\"content\":{\"connectorIds\":[],\"side\":\"BOTTOM\"},\"type\":\"ConnectorPlacement.EquallySpacedRectSide\",\"uuid\":\"853ec498-094f-4e09-abd5-bb70086bab7d\"}]},\"type\":\"ConnectorPlacement.EquallySpacedConnector\",\"uuid\":\"f62687dc-336d-43b3-90e2-c71aecc80de5\"}],\"packageUris\":[\"http://schema.mathworks.com/mf0/Connector/R2020b\"],\"version\":\"1.0\"}"
  F5.5 Move the Gripper towards Product : Subsystem
      settings: PortSchema="{\"entries\":[{\"content\":{\"headerSize\":26,\"margin\":15,\"minimumSpacing\":25,\"sides\":[{\"content\":{\"connectorIds\":[\"In1\"]},\"type\":\"ConnectorPlacement.EquallySpacedRectSide\",\"uuid\":\"ce520cb7-ac6b-49f5-959a-43d0066e6af8\"},{\"content\":{\"connectorIds\":[\"Out1\"],\"side\":\"RIGHT\"},\"type\":\"ConnectorPlacement.EquallySpacedRectSide\",\"uuid\":\"785c5fb5-eec3-4a9f-be3c-47cdb1865e9b\"},{\"content\":{\"connectorIds\":[],\"side\":\"TOP\"},\"type\":\"ConnectorPlacement.EquallySpacedRectSide\",\"uuid\":\"de1fb606-e36e-4d03-b808-745512e6c407\"}]},\"type\":\"ConnectorPlacement.EquallySpacedConnector\",\"uuid\":\"f62687dc-336d-43b3-90e2-c71aecc80de5\"}],\"packageUris\":[\"http://schema.mathworks.com/mf0/Connector/R2020b\"],\"version\":\"1.0\"}"
  F5.6 Activate Gripper : Subsystem
      settings: PortSchema="{\"entries\":[{\"content\":{\"headerSize\":26,\"margin\":15,\"minimumSpacing\":25,\"sides\":[{\"content\":{\"connectorIds\":[\"In1\",\"In2\"]},\"type\":\"ConnectorPlacement.EquallySpacedRectSide\",\"uuid\":\"ce520cb7-ac6b-49f5-959a-43d0066e6af8\"},{\"content\":{\"connectorIds\":[\"Out2\"],\"side\":\"RIGHT\"},\"type\":\"ConnectorPlacement.EquallySpacedRectSide\",\"uuid\":\"785c5fb5-eec3-4a9f-be3c-47cdb1865e9b\"},{\"content\":{\"connectorIds\":[\"Out1\"],\"side\":\"TOP\"},\"type\":\"ConnectorPlacement.EquallySpacedRectSide\",\"uuid\":\"de1fb606-e36e-4d03-b808-745512e6c407\"}]},\"type\":\"ConnectorPlacement.EquallySpacedConnector\",\"uuid\":\"f62687dc-336d-43b3-90e2-c71aecc80de5\"}],\"packageUris\":[\"http://schema.mathworks.com/mf0/Connector/R2020b\"],\"version\":\"1.0\"}"
  Bus Element Out3 : Outport  PortName=Current Position
  Bus Element Out4 : Outport  Port=2  PortName=Current Force
  Bus Element Out1 : Outport  Port=3  PortName=Product Picked
  wires:
  F5.4 Check and Verify Force and Position of Gripper/1(New Force value) -> F5.6 Activate Gripper/1(New Force value)
  Bus Element In2/1 -> F5.4 Check and Verify Force and Position of Gripper/1(Corrected Force)
  Bus Element In3/1 -> F5.4 Check and Verify Force and Position of Gripper/2(Corrected Postition)
  F5.1 Accept Coordinates/1(Importedcoordiantes) -> F5.3 Compute Trajectory/2(Importedcoordinates)
  F5.4 Check and Verify Force and Position of Gripper/2(New coordinates) -> F5.3 Compute Trajectory/1(New coordinates)
  F5.2 Import Orientation of Product/1(Importedorientation) -> F5.3 Compute Trajectory/3(Importedorientation)
  F5.3 Compute Trajectory/2(Defined Path) -> F5.5 Move the Gripper towards Product/1(Defined Path)
  F5.5 Move the Gripper towards Product/1(Ready to pick Pick Product) -> F5.6 Activate Gripper/2(Ready to pick Pick Product)
  F5.6 Activate Gripper/2(Product Picked) -> Bus Element Out1/1
  Begin Task/1(Coordinates) -> F5.1 Accept Coordinates/1(Coordinates)
  Begin Task/2(Orientation) -> F5.2 Import Orientation of Product/1(Orientation)
  Bus Element In4/1 -> Begin Task/1(Beiginpickoperation)
  F5.3 Compute Trajectory/1(Current Position) -> Bus Element Out3/1
  F5.6 Activate Gripper/1(Current Force) -> Bus Element Out4/1

== system System_composer__model_pre_alpha_V2/Actuate Robot/StopSignalisFalse/F6 Translate Product ==
  Bus Element In1 : Inport  PortName=Product Picked
  F6.1 Move : Subsystem
      settings: PortSchema="{\"entries\":[{\"content\":{\"headerSize\":26,\"margin\":15,\"minimumSpacing\":25,\"sides\":[{\"content\":{\"connectorIds\":[\"In1\"]},\"type\":\"ConnectorPlacement.EquallySpacedRectSide\",\"uuid\":\"ce520cb7-ac6b-49f5-959a-43d0066e6af8\"},{\"content\":{\"connectorIds\":[\"Out1\"],\"side\":\"RIGHT\"},\"type\":\"ConnectorPlacement.EquallySpacedRectSide\",\"uuid\":\"785c5fb5-eec3-4a9f-be3c-47cdb1865e9b\"},{\"content\":{\"connectorIds\":[],\"side\":\"TOP\"},\"type\":\"ConnectorPlacement.EquallySpacedRectSide\",\"uuid\":\"de1fb606-e36e-4d03-b808-745512e6c407\"}]},\"type\":\"ConnectorPlacement.EquallySpacedConnector\",\"uuid\":\"f62687dc-336d-43b3-90e2-c71aecc80de5\"}],\"packageUris\":[\"http://schema.mathworks.com/mf0/Connector/R2020b\"],\"version\":\"1.0\"}"
  Bus Element Out1 : Outport  PortName=Ready to be Placed
  wires:
  Bus Element In1/1 -> F6.1 Move/1(Product Picked)
  F6.1 Move/1(Ready to be Placed) -> Bus Element Out1/1

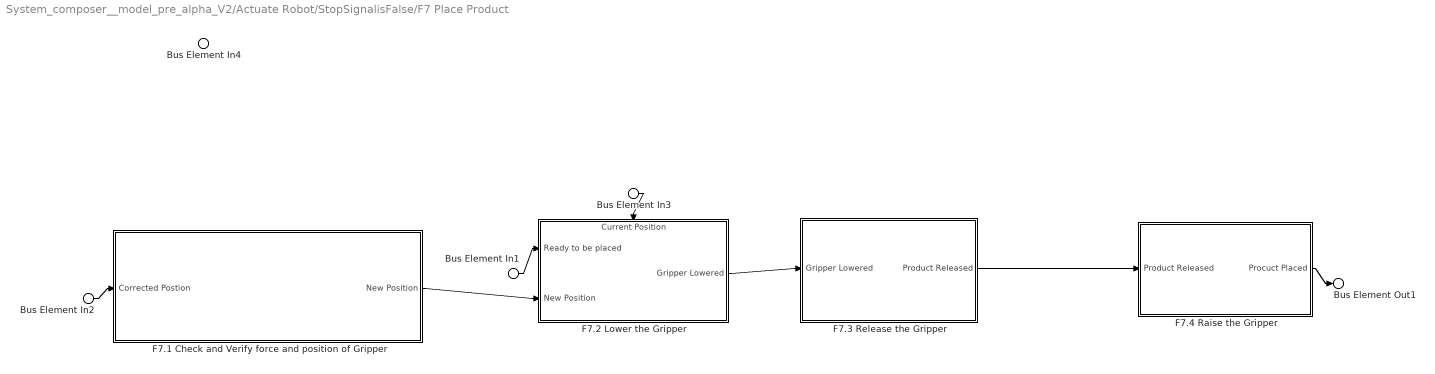
== system System_composer__model_pre_alpha_V2/Actuate Robot/StopSignalisFalse/F7 Place Product ==
  Bus Element In4 : Inport  PortName=InBus
  Bus Element In3 : Inport  Port=2  PortName=Current Position
  Bus Element In1 : Inport  Port=3  PortName=Ready to be placed
  Bus Element In2 : Inport  Port=4  PortName=Corrected Postion
  F7.1 Check and Verify force and position of Gripper : Subsystem
      settings: PortSchema="{\"entries\":[{\"content\":{\"headerSize\":26,\"margin\":15,\"minimumSpacing\":25,\"sides\":[{\"content\":{\"connectorIds\":[\"In1\"]},\"type\":\"ConnectorPlacement.EquallySpacedRectSide\",\"uuid\":\"ce520cb7-ac6b-49f5-959a-43d0066e6af8\"},{\"content\":{\"connectorIds\":[\"Out1\"],\"side\":\"RIGHT\"},\"type\":\"ConnectorPlacement.EquallySpacedRectSide\",\"uuid\":\"785c5fb5-eec3-4a9f-be3c-47cdb1865e9b\"},{\"content\":{\"connectorIds\":[],\"side\":\"TOP\"},\"type\":\"ConnectorPlacement.EquallySpacedRectSide\",\"uuid\":\"de1fb606-e36e-4d03-b808-745512e6c407\"}]},\"type\":\"ConnectorPlacement.EquallySpacedConnector\",\"uuid\":\"f62687dc-336d-43b3-90e2-c71aecc80de5\"}],\"packageUris\":[\"http://schema.mathworks.com/mf0/Connector/R2020b\"],\"version\":\"1.0\"}"
  F7.2 Lower the Gripper : Subsystem
      settings: PortSchema="{\"entries\":[{\"content\":{\"headerSize\":26,\"margin\":15,\"minimumSpacing\":25,\"sides\":[{\"content\":{\"connectorIds\":[\"In2\",\"In3\"]},\"type\":\"ConnectorPlacement.EquallySpacedRectSide\",\"uuid\":\"ce520cb7-ac6b-49f5-959a-43d0066e6af8\"},{\"content\":{\"connectorIds\":[\"Out1\"],\"side\":\"RIGHT\"},\"type\":\"ConnectorPlacement.EquallySpacedRectSide\",\"uuid\":\"785c5fb5-eec3-4a9f-be3c-47cdb1865e9b\"},{\"content\":{\"connectorIds\":[\"In1\"],\"side\":\"TOP\"},\"type\":\"ConnectorPlacement.EquallySpacedRectSide\",\"uuid\":\"de1fb606-e36e-4d03-b808-745512e6c407\"}]},\"type\":\"ConnectorPlacement.EquallySpacedConnector\",\"uuid\":\"f62687dc-336d-43b3-90e2-c71aecc80de5\"}],\"packageUris\":[\"http://schema.mathworks.com/mf0/Connector/R2020b\"],\"version\":\"1.0\"}"
  F7.3 Release the Gripper : Subsystem
      settings: PortSchema="{\"entries\":[{\"content\":{\"headerSize\":26,\"margin\":15,\"minimumSpacing\":25,\"sides\":[{\"content\":{\"connectorIds\":[\"In1\"]},\"type\":\"ConnectorPlacement.EquallySpacedRectSide\",\"uuid\":\"ce520cb7-ac6b-49f5-959a-43d0066e6af8\"},{\"content\":{\"connectorIds\":[\"Out1\"],\"side\":\"RIGHT\"},\"type\":\"ConnectorPlacement.EquallySpacedRectSide\",\"uuid\":\"785c5fb5-eec3-4a9f-be3c-47cdb1865e9b\"},{\"content\":{\"connectorIds\":[],\"side\":\"TOP\"},\"type\":\"ConnectorPlacement.EquallySpacedRectSide\",\"uuid\":\"de1fb606-e36e-4d03-b808-745512e6c407\"}]},\"type\":\"ConnectorPlacement.EquallySpacedConnector\",\"uuid\":\"f62687dc-336d-43b3-90e2-c71aecc80de5\"}],\"packageUris\":[\"http://schema.mathworks.com/mf0/Connector/R2020b\"],\"version\":\"1.0\"}"
  F7.4 Raise the Gripper : Subsystem
      settings: PortSchema="{\"entries\":[{\"content\":{\"headerSize\":26,\"margin\":15,\"minimumSpacing\":25,\"sides\":[{\"content\":{\"connectorIds\":[\"In1\"]},\"type\":\"ConnectorPlacement.EquallySpacedRectSide\",\"uuid\":\"ce520cb7-ac6b-49f5-959a-43d0066e6af8\"},{\"content\":{\"connectorIds\":[\"Out1\"],\"side\":\"RIGHT\"},\"type\":\"ConnectorPlacement.EquallySpacedRectSide\",\"uuid\":\"785c5fb5-eec3-4a9f-be3c-47cdb1865e9b\"},{\"content\":{\"connectorIds\":[],\"side\":\"TOP\"},\"type\":\"ConnectorPlacement.EquallySpacedRectSide\",\"uuid\":\"de1fb606-e36e-4d03-b808-745512e6c407\"}]},\"type\":\"ConnectorPlacement.EquallySpacedConnector\",\"uuid\":\"f62687dc-336d-43b3-90e2-c71aecc80de5\"}],\"packageUris\":[\"http://schema.mathworks.com/mf0/Connector/R2020b\"],\"version\":\"1.0\"}"
  Bus Element Out1 : Outport  PortName=Product Placed
  wires:
  F7.4 Raise the Gripper/1(Procuct Placed) -> Bus Element Out1/1
  Bus Element In1/1 -> F7.2 Lower the Gripper/2(Ready to be placed)
  Bus Element In2/1 -> F7.1 Check and Verify force and position of Gripper/1(Corrected Postion)
  F7.1 Check and Verify force and position of Gripper/1(New Position) -> F7.2 Lower the Gripper/3(New Position)
  F7.2 Lower the Gripper/1(Gripper Lowered) -> F7.3 Release the Gripper/1(Gripper Lowered)
  F7.3 Release the Gripper/1(Product Released) -> F7.4 Raise the Gripper/1(Product Released)
  Bus Element In3/1 -> F7.2 Lower the Gripper/1(Current Position)

== system System_composer__model_pre_alpha_V2/F2 Inspect Product/Compute dimentions of product/Compute dimention ==
  Bus Element In1 : Inport  PortName=Coordinates
  Bus Element Out1 : Outport  PortName=Dimention of product

== system System_composer__model_pre_alpha_V2/F2 Inspect Product/Compute dimentions of product/get coordinates ==
  Bus Element In1 : Inport  PortName=Product image
  Bus Element Out1 : Outport  PortName=Coordinates

== system System_composer__model_pre_alpha_V2/F4 Calibrate Systems /Physical setup/Frame setup ==
  Bus Element In1 : Inport  PortName=Frame components
  Bus Element Out1 : Outport  PortName=Frame

== system System_composer__model_pre_alpha_V2/F4 Calibrate Systems /Physical setup/Motor setup ==
  Bus Element In1 : Inport  PortName=Frame
  Bus Element In2 : Inport  Port=2  PortName=Motor
  Bus Element Out1 : Outport  PortName=Frame and motor setup

== system System_composer__model_pre_alpha_V2/F4 Calibrate Systems /Physical setup/Power upset ==
  Bus Element In2 : Inport  PortName=Power
  Bus Element In1 : Inport  Port=2  PortName=Frame and motor setup
  Bus Element Out1 : Outport  PortName=Physical setup

== system System_composer__model_pre_alpha_V2/Actuate Robot/StopSignalisFalse/F08 Handle Contingencies/Check Pick Position ==
  Position of gripper : Inport
  Around the specified area : Subsystem  VariantControl=true
      settings: PortSchema="{\"entries\":[{\"content\":{\"headerSize\":26,\"margin\":15,\"minimumSpacing\":25,\"sides\":[{\"content\":{\"connectorIds\":[]},\"type\":\"ConnectorPlacement.EquallySpacedRectSide\",\"uuid\":\"7245304e-b65d-462b-853e-3a80a6fffb1c\"},{\"content\":{\"connectorIds\":[\"Out1\"],\"side\":\"RIGHT\"},\"type\":\"ConnectorPlacement.EquallySpacedRectSide\",\"uuid\":\"9267bc47-a16a-4902-a507-692f8de66c88\"},{\"content\":{\"connectorIds\":[],\"side\":\"TOP\"},\"type\":\"ConnectorPlacement.EquallySpacedRectSide\",\"uuid\":\"a6bb1c3e-d38e-4cbb-9a53-bfb7d2a1449e\"}]},\"type\":\"ConnectorPlacement.EquallySpacedConnector\",\"uuid\":\"8b606370-32fa-4262-8c68-990651fac4cc\"}],\"packageUris\":[\"http://schema.mathworks.com/mf0/Connector/R2020b\"],\"version\":\"1.0\"}"
  Beyond the range : Subsystem  VariantControl=Choice
      settings: PortSchema="{\"entries\":[{\"content\":{\"headerSize\":26,\"margin\":15,\"minimumSpacing\":25,\"sides\":[{\"content\":{\"connectorIds\":[]},\"type\":\"ConnectorPlacement.EquallySpacedRectSide\",\"uuid\":\"cfa9a458-ccb1-4b4b-9223-cdb6aaef5fc4\"},{\"content\":{\"connectorIds\":[],\"side\":\"RIGHT\"},\"type\":\"ConnectorPlacement.EquallySpacedRectSide\",\"uuid\":\"f9e6f688-270f-46a5-8c07-32c6831cf3d3\"},{\"content\":{\"connectorIds\":[],\"side\":\"TOP\"},\"type\":\"ConnectorPlacement.EquallySpacedRectSide\",\"uuid\":\"2fcd258a-a10a-44a0-bcb2-682252ae81b0\"}]},\"type\":\"ConnectorPlacement.EquallySpacedConnector\",\"uuid\":\"80e45476-3fa2-42b9-aef1-d9f502108577\"}],\"packageUris\":[\"http://schema.mathworks.com/mf0/Connector/R2020b\"],\"version\":\"1.0\"}"
  Corrected position : Outport

== system System_composer__model_pre_alpha_V2/Actuate Robot/StopSignalisFalse/F08 Handle Contingencies/F8.1Weak force on the product ==
  Bus Element In1 : Inport  PortName=Force on gripper
  Bus Element Out1 : Outport  PortName=Appropriate force

== system System_composer__model_pre_alpha_V2/Actuate Robot/StopSignalisFalse/F5 Pick Product/Begin Task ==
  Bus Element In1 : Inport  PortName=Beiginpickoperation
  Bus Element Out1 : Outport  PortName=Coordinates
  Bus Element Out2 : Outport  Port=2  PortName=Orientation

== system System_composer__model_pre_alpha_V2/Actuate Robot/StopSignalisFalse/F5 Pick Product/F5.1 Accept Coordinates ==
  Bus Element In1 : Inport  PortName=Coordinates
  Bus Element Out1 : Outport  PortName=Importedcoordiantes
